simulink model "Vehicle_Radar_Model"  (R2013a)
settings: Solver=ode4  StartTime=0.0  StopTime=100  FixedStep=0.001  MaxStep=0.001  RelTol=1e-3
model workspace (MAT data in the model file):
  Fy_Angle = [-20; -16; -14; -12; -10; -9.5; -9; -8.5; -8; -7.5; -7; -6.5; -6; -5.5; -5; -4.5; -4; -3.5; -3; -2.5; -2; -1.5; -1; -0.5; 0; 0.5; 1; 1.5; 2; 2.5; 3; 3.5; 4; 4.5; 5; 5.5; 6; 6.5; 7; 7.5; 8; 8.5; 9; 9.5; 10; 12; 14; 16; 18; 20]
  Fy_W = [1725 3500 6100 6950 9005]
  Fy_Data = [-1523.64 -1531.91 -1546.58 -1574.53 -1631.62 -1653.27 -1678.67 -1707.8 -1740.18 -1775.12 -1810.95 -1845.3 ... (250 elements, 50x5)]
  Cr = 38255
  Cf = 38925
  lr = 1.6662
  Izz = 4192
  lf = 1.11
  m = 1530
  GearRatio = 17.25
  Pb2Tq_r = 150
  Pb2Tq_f = 300
  t2e = 2000
  R_Tire = 0.33
  Iyy_Tire = 0.9
  Fx_SL = [-1; -0.9; -0.8; -0.7; -0.6; -0.5; -0.4; -0.3; -0.25; -0.2; -0.18; -0.16; -0.14; -0.12; -0.1; -0.08; -0.06; -0.04; -0.02; 0; 0.02; 0.04; 0.06; 0.08; 0.1; 0.12; 0.14; 0.16; 0.18; 0.2; 0.25; 0.3; 0.4; 0.5; 0.6; 0.7; 0.8; 0.9; 1]
  Fx_W = [2105 3995 6120 7900 10100]
  Fx_Data = [-2029.26  -4058.51  -6087.76  -8117.01  -10146.3; -2029.26  -4058.51  -6087.76  -8117.01  -10146.3; -2053.55  -4107.12  -6160.67  -8214.24  -10267.8; -2084.58  -4169.16  -6253.75  -8338.33  -10422.9; -2125.47  -4250.95  -6376.42  -8501.91  -10627.4; -2181.64  -4363.28  -6544.93  -8726.56  -10908.2; -2262.94  -4525.87  -6788.82  -9051.76  -11314.7; -2388.22  -4776.46  -7164.69  -9552.92  -11941.1; -2476.95  -4953.9  -7430.85  -9907.79  -12384.7; -2586.89  -5173.78  -7760.68  -10347.6  -12934.4; -2634.75  -5269.5  -7904.24  -10539  -13173.7; -2680.7  -5361.4  -8042.1  -10722.8  -13403.5; -2717.36  -5434.73  -8152.09  -10869.4  -13586.8; -2729.82  -5459.63  -8189.45  -10919.3  -13649.1; -2689.78  -5379.54  -8069.32  -10759.1  -13448.8; -2548.95  -5097.92  -7646.88  -10195.8  -12744.8; -2240.07  -4480.13  -6720.21  -8960.27  -11200.3; -1701.43  -3402.86  -5104.29  -6805.72  -8507.15; -926.741  -1853.48  -2780.22  -3706.97  -4633.7; 0  0  0  0  0; 926.741  1853.48  2780.22  3706.97  4633.7; 1701.43  3402.86  5104.29  6805.72  8507.15; 2240.07  4480.13  6720.21  8960.27  11200.3; 2548.95  5097.92  7646.88  10195.8  12744.8; 2689.78  5379.54  8069.32  10759.1  13448.8; 2729.82  5459.63  8189.45  10919.3  13649.1; 2717.36  5434.73  8152.09  10869.4  13586.8; 2680.7  5361.4  8042.1  10722.8  13403.5; 2634.75  5269.5  7904.24  10539  13173.7; 2586.89  5173.78  7760.68  10347.6  12934.4; 2476.95  4953.9  7430.85  9907.79  12384.7; 2388.22  4776.46  7164.69  9552.92  11941.1; 2262.94  4525.87  6788.82  9051.76  11314.7; 2181.64  4363.28  6544.93  8726.56  10908.2; 2125.47  4250.95  6376.42  8501.91  10627.4; 2084.58  4169.16  6253.75  8338.33  10422.9; 2053.55  4107.12  6160.67  8214.24  10267.8; 2029.26  4058.51  6087.76  8117.01  10146.3; 2029.26  4058.51  6087.76  8117.01  10146.3]
  g = 9.81
  K = 19
  mu = 0.9
libraries: simulink x1
settings Model: Creator=Park  LastModifiedBy=IVDL
settings DataIOCC: LimitDataPoints=off  SignalLoggingSaveFormat=ModelDataLogs
settings OptimizationCC: ExpressionDepthLimit=2147483647
settings DebuggingCC: MultiTaskDSMMsg=warning  MultiTaskCondExecSysMsg=none  FcnCallInpInsideContextMsg=UseLocalSettings  StrictBusMsg=None
settings RTWCC: IncludeERTFirstTime=on
settings GRTTargetCC: CodeReplacementLibrary=None  CombineOutputUpdateFcns=off  CPPClassGenCompliant=on  GRTInterface=on

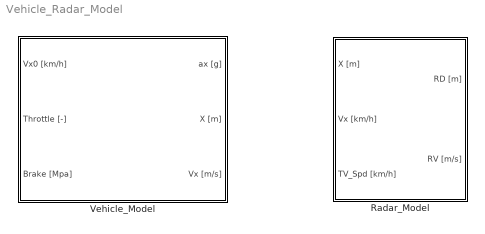
== system Vehicle_Radar_Model ==
  Radar_Model : Subsystem
  Vehicle_Model : Subsystem

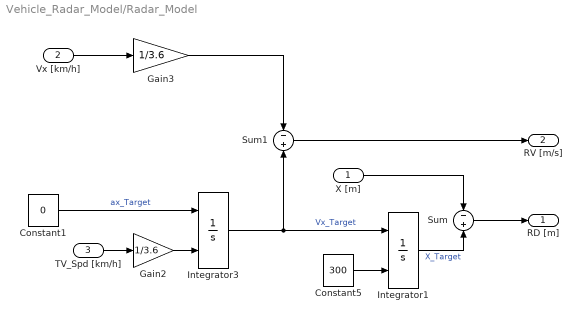
== system Vehicle_Radar_Model/Radar_Model ==
  X [m] : Inport
  Vx [km/h] : Inport  Port=2
  TV_Spd [km/h] : Inport  Port=3
  Constant1 : Constant  Value=0
  Constant5 : Constant  Value=300
  Gain2 : Gain  Gain=1/3.6
  Gain3 : Gain  Gain=1/3.6
  Integrator1 : Integrator  InitialConditionSource=external  InitialCondition=500
  Integrator3 : Integrator  InitialConditionSource=external  InitialCondition=80  LimitOutput=on  LowerSaturationLimit=0
  Sum : Sum  Inputs=-+
  Sum1 : Sum  Inputs=-+
  RD [m] : Outport
  RV [m/s] : Outport  Port=2
  wires:
  TV_Spd [km/h]/1 -> Gain2/1
  Constant1/1 -> Integrator3/1  "ax_Target"
  Integrator3/1 -> Integrator1/1, Sum1/2  "Vx_Target"
  Integrator1/1 -> Sum/2  "X_Target"
  Constant5/1 -> Integrator1/2
  Sum/1 -> RD [m]/1
  X [m]/1 -> Sum/1
  Vx [km/h]/1 -> Gain3/1
  Sum1/1 -> RV [m/s]/1
  Gain2/1 -> Integrator3/2
  Gain3/1 -> Sum1/1

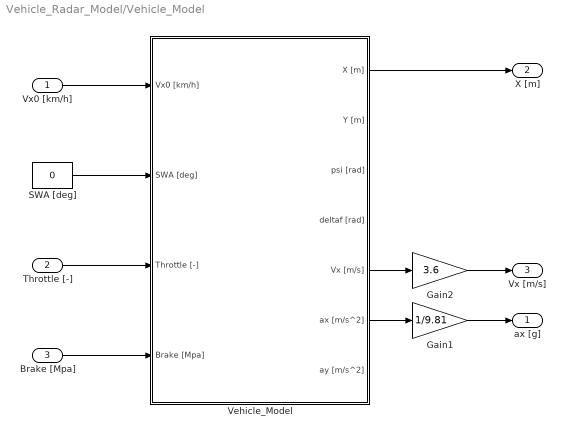
== system Vehicle_Radar_Model/Vehicle_Model ==
  Vx0 [km/h] : Inport
  Throttle [-] : Inport  Port=2
  Brake [Mpa] : Inport  Port=3
  Gain1 : Gain  Gain=1/9.81
  Gain2 : Gain  Gain=3.6
  SWA [deg] : Constant  Value=0
  Vehicle_Model : Subsystem
  ax [g] : Outport
  X [m] : Outport  Port=2
  Vx [m/s] : Outport  Port=3
  wires:
  Gain1/1 -> ax [g]/1
  Gain2/1 -> Vx [m/s]/1
  Vehicle_Model/1(X [m]) -> X [m]/1
  Throttle [-]/1 -> Vehicle_Model/3(Throttle [-])
  Brake [Mpa]/1 -> Vehicle_Model/4(Brake [Mpa])
  Vehicle_Model/6(ax [m/s^2]) -> Gain1/1
  Vehicle_Model/5(Vx [m/s]) -> Gain2/1
  SWA [deg]/1 -> Vehicle_Model/2(SWA [deg])
  Vx0 [km/h]/1 -> Vehicle_Model/1(Vx0 [km/h])

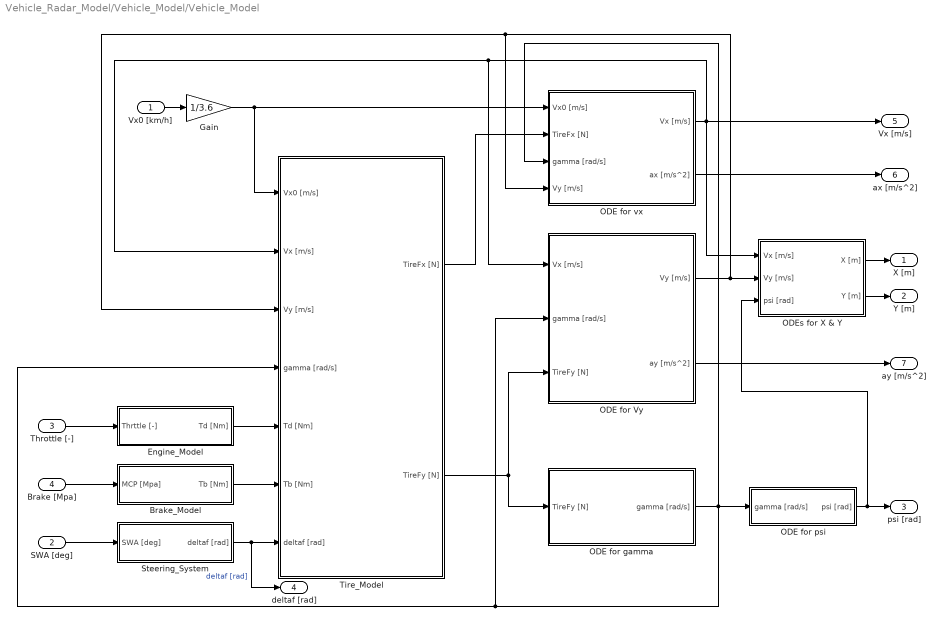
== system Vehicle_Radar_Model/Vehicle_Model/Vehicle_Model ==
  Vx0 [km/h] : Inport
  SWA [deg] : Inport  Port=2
  Throttle [-] : Inport  Port=3
  Brake [Mpa] : Inport  Port=4
  Brake_Model : Subsystem
  Engine_Model : Subsystem
  Gain : Gain  Gain=1/3.6
  ODE for Vy : Subsystem
  ODE for gamma : Subsystem
  ODE for psi : Subsystem
  ODE for vx : Subsystem
  ODEs for X & Y : Subsystem
  Steering_System : Subsystem
  Tire_Model : Subsystem
  X [m] : Outport
  Y [m] : Outport  Port=2
  psi [rad] : Outport  Port=3
  deltaf [rad] : Outport  Port=4
  Vx [m/s] : Outport  Port=5
  ax [m/s^2] : Outport  Port=6
  ay [m/s^2] : Outport  Port=7
  wires:
  ODE for Vy/2(ay [m/s^2]) -> ay [m/s^2]/1
  ODE for vx/2(ax [m/s^2]) -> ax [m/s^2]/1
  ODEs for X & Y/2(Y [m]) -> Y [m]/1
  ODEs for X & Y/1(X [m]) -> X [m]/1
  ODE for psi/1(psi [rad]) -> ODEs for X & Y/3(psi [rad]), psi [rad]/1
  ODE for Vy/1(Vy [m/s]) -> ODEs for X & Y/2(Vy [m/s]), Tire_Model/3(Vy [m/s]), ODE for vx/4(Vy [m/s])
  ODE for gamma/1(gamma [rad/s]) -> ODE for Vy/2(gamma [rad/s]), Tire_Model/4(gamma [rad/s]), ODE for psi/1(gamma [rad/s]), ODE for vx/3(gamma [rad/s])
  Tire_Model/2(TireFy [N]) -> ODE for gamma/1(TireFy [N]), ODE for Vy/3(TireFy [N])
  ODE for vx/1(Vx [m/s]) -> Tire_Model/2(Vx [m/s]), ODE for Vy/1(Vx [m/s]), ODEs for X & Y/1(Vx [m/s]), Vx [m/s]/1
  Steering_System/1(deltaf [rad]) -> Tire_Model/7(deltaf [rad]), deltaf [rad]/1  "deltaf [rad]"
  Tire_Model/1(TireFx [N]) -> ODE for vx/2(TireFx [N])
  Throttle [-]/1 -> Engine_Model/1(Thrttle [-])
  Brake [Mpa]/1 -> Brake_Model/1(MCP [Mpa])
  Brake_Model/1(Tb [Nm]) -> Tire_Model/6(Tb [Nm])
  Engine_Model/1(Td [Nm]) -> Tire_Model/5(Td [Nm])
  Gain/1 -> Tire_Model/1(Vx0 [m/s]), ODE for vx/1(Vx0 [m/s])
  SWA [deg]/1 -> Steering_System/1(SWA [deg])
  Vx0 [km/h]/1 -> Gain/1

== system Vehicle_Radar_Model/Vehicle_Model/Vehicle_Model/Brake_Model ==
  MCP [Mpa] : Inport
  Gain : Gain  Gain=2*Pb2Tq_f
  Gain1 : Gain  Gain=2*Pb2Tq_r
  Mux : Mux  Inputs=2
  Transfer Fcn : TransferFcn  Denominator=[0.06 1]
  Transfer Fcn1 : TransferFcn  Denominator=[0.06 1]
  Tb [Nm] : Outport
  wires:
  Transfer Fcn1/1 -> Mux/2
  Transfer Fcn/1 -> Mux/1
  Mux/1 -> Tb [Nm]/1
  MCP [Mpa]/1 -> Gain/1, Gain1/1
  Gain1/1 -> Transfer Fcn1/1  "Tb_r [Nm]"
  Gain/1 -> Transfer Fcn/1  "Tb_f [Nm]"

== system Vehicle_Radar_Model/Vehicle_Model/Vehicle_Model/Engine_Model ==
  Thrttle [-] : Inport
  Gain : Gain  Gain=t2e
  Transfer Fcn : TransferFcn  Numerator=[100]  Denominator=[1 2*0.5*10 100]
  Td [Nm] : Outport
  wires:
  Transfer Fcn/1 -> Td [Nm]/1
  Gain/1 -> Transfer Fcn/1
  Thrttle [-]/1 -> Gain/1

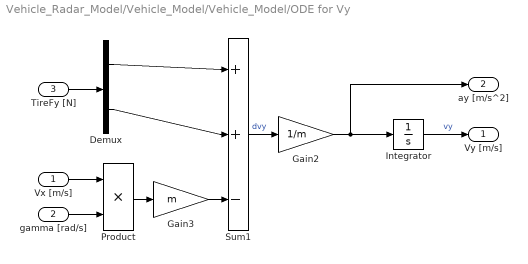
== system Vehicle_Radar_Model/Vehicle_Model/Vehicle_Model/ODE for Vy ==
  Vx [m/s] : Inport
  gamma [rad/s] : Inport  Port=2
  TireFy [N] : Inport  Port=3
  Demux : Demux  Outputs=2
  Gain2 : Gain  Gain=1/m
  Gain3 : Gain  Gain=m
  Integrator : Integrator
  Product : Product  RndMeth=Zero
  Sum1 : Sum  Inputs=++|-
  Vy [m/s] : Outport
  ay [m/s^2] : Outport  Port=2
  wires:
  Gain2/1 -> Integrator/1, ay [m/s^2]/1
  Gain3/1 -> Sum1/3
  TireFy [N]/1 -> Demux/1
  gamma [rad/s]/1 -> Product/2
  Vx [m/s]/1 -> Product/1
  Integrator/1 -> Vy [m/s]/1  "vy"
  Product/1 -> Gain3/1
  Sum1/1 -> Gain2/1  "dvy"
  Demux/2 -> Sum1/2
  Demux/1 -> Sum1/1

== system Vehicle_Radar_Model/Vehicle_Model/Vehicle_Model/ODE for gamma ==
  TireFy [N] : Inport
  Demux : Demux  Outputs=2
  Gain4 : Gain  Gain=1/Izz
  Gain5 : Gain  Gain=lf
  Gain6 : Gain  Gain=lr
  Integrator2 : Integrator
  Sum2 : Sum  Inputs=+-
  gamma [rad/s] : Outport
  wires:
  TireFy [N]/1 -> Demux/1
  Demux/2 -> Gain6/1
  Integrator2/1 -> gamma [rad/s]/1  "gamma"
  Demux/1 -> Gain5/1
  Gain6/1 -> Sum2/2
  Gain5/1 -> Sum2/1
  Gain4/1 -> Integrator2/1
  Sum2/1 -> Gain4/1

== system Vehicle_Radar_Model/Vehicle_Model/Vehicle_Model/ODE for psi ==
  gamma [rad/s] : Inport
  Integrator : Integrator  ContinuousStateAttributes='psi'
  psi [rad] : Outport
  wires:
  gamma [rad/s]/1 -> Integrator/1  "dpsi"
  Integrator/1 -> psi [rad]/1

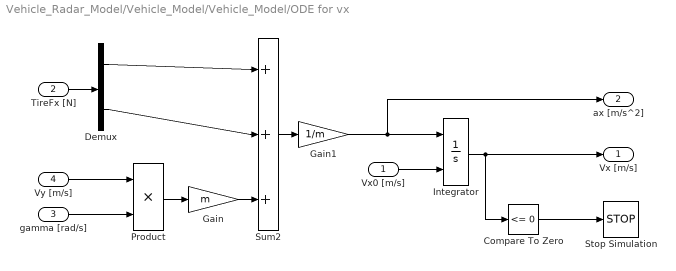
== system Vehicle_Radar_Model/Vehicle_Model/Vehicle_Model/ODE for vx ==
  Vx0 [m/s] : Inport
  TireFx [N] : Inport  Port=2
  gamma [rad/s] : Inport  Port=3
  Vy [m/s] : Inport  Port=4
  Compare To Zero : simulink/Logic and Bit Operations/Compare To Zero  relop=<=  OutDataTypeStr=boolean
  Demux : Demux  Outputs=2
  Gain : Gain  Gain=m
  Gain1 : Gain  Gain=1/m
  Integrator : Integrator  InitialConditionSource=external
  Product : Product  RndMeth=Zero
  Stop Simulation : Stop
  Sum2 : Sum  Inputs=++|+
  Vx [m/s] : Outport
  ax [m/s^2] : Outport  Port=2
  wires:
  Gain1/1 -> Integrator/1, ax [m/s^2]/1
  Compare To Zero/1 -> Stop Simulation/1
  Gain/1 -> Sum2/3
  Product/1 -> Gain/1
  Sum2/1 -> Gain1/1
  gamma [rad/s]/1 -> Product/2
  Vy [m/s]/1 -> Product/1
  Demux/2 -> Sum2/2
  Demux/1 -> Sum2/1
  TireFx [N]/1 -> Demux/1
  Integrator/1 -> Vx [m/s]/1, Compare To Zero/1
  Vx0 [m/s]/1 -> Integrator/2

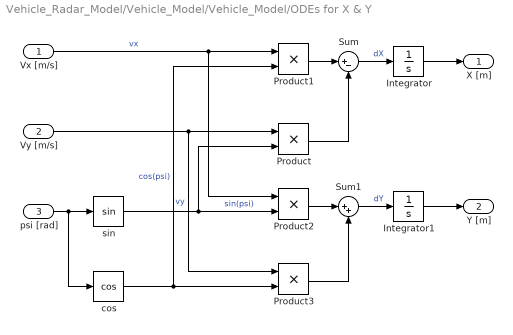
== system Vehicle_Radar_Model/Vehicle_Model/Vehicle_Model/ODEs for X & Y ==
  Vx [m/s] : Inport
  Vy [m/s] : Inport  Port=2
  psi [rad] : Inport  Port=3
  Integrator : Integrator  ContinuousStateAttributes='X'
  Integrator1 : Integrator  ContinuousStateAttributes='Y'
  Product{,1..3} (4 alike) : Product  RndMeth=Zero
  Sum : Sum  Inputs=|+-
  Sum1 : Sum  Inputs=|++
  cos : Trigonometry  Operator=cos
  sin : Trigonometry
  X [m] : Outport
  Y [m] : Outport  Port=2
  wires:
  Integrator1/1 -> Y [m]/1
  Integrator/1 -> X [m]/1
  Sum1/1 -> Integrator1/1  "dY"
  Product3/1 -> Sum1/2
  Product2/1 -> Sum1/1
  Sum/1 -> Integrator/1  "dX"
  Product/1 -> Sum/2
  Product1/1 -> Sum/1
  cos/1 -> Product3/2, Product1/2  "cos(psi)"
  Vx [m/s]/1 -> Product2/1, Product1/1  "vx"
  Vy [m/s]/1 -> Product3/1, Product/1  "vy"
  sin/1 -> Product2/2, Product/2  "sin(psi)"
  psi [rad]/1 -> cos/1, sin/1

== system Vehicle_Radar_Model/Vehicle_Model/Vehicle_Model/Steering_System ==
  SWA [deg] : Inport
  Gain : Gain  Gain=1/GearRatio
  Gain5 : Gain  Gain=pi/180
  Saturation : Saturate  UpperLimit=540  LowerLimit=-540
  deltaf [rad] : Outport
  wires:
  Saturation/1 -> Gain/1
  SWA [deg]/1 -> Saturation/1
  Gain5/1 -> deltaf [rad]/1
  Gain/1 -> Gain5/1

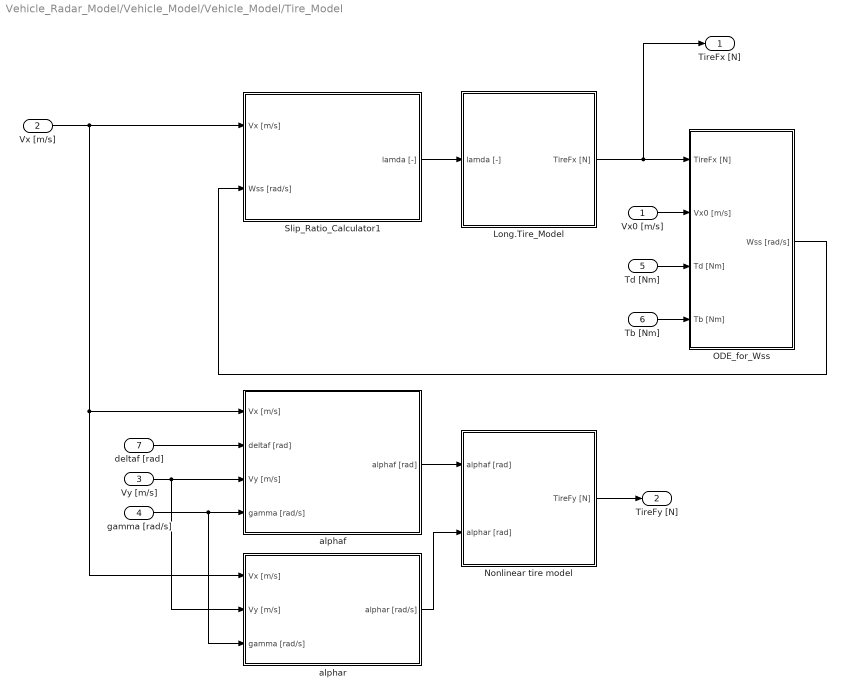
== system Vehicle_Radar_Model/Vehicle_Model/Vehicle_Model/Tire_Model ==
  Vx0 [m/s] : Inport
  Vx [m/s] : Inport  Port=2
  Vy [m/s] : Inport  Port=3
  gamma [rad/s] : Inport  Port=4
  Td [Nm] : Inport  Port=5
  Tb [Nm] : Inport  Port=6
  deltaf [rad] : Inport  Port=7
  Long.Tire_Model : Subsystem
  Nonlinear tire model : Subsystem
  ODE_for_Wss : Subsystem
  Slip_Ratio_Calculator1 : Subsystem
  alphaf : Subsystem
  alphar : Subsystem
  TireFx [N] : Outport
  TireFy [N] : Outport  Port=2
  wires:
  Nonlinear tire model/1(TireFy [N]) -> TireFy [N]/1
  gamma [rad/s]/1 -> alphaf/4(gamma [rad/s]), alphar/3(gamma [rad/s])
  Vy [m/s]/1 -> alphar/2(Vy [m/s]), alphaf/3(Vy [m/s])
  deltaf [rad]/1 -> alphaf/2(deltaf [rad])
  alphar/1(alphar [rad/s]) -> Nonlinear tire model/2(alphar [rad])
  alphaf/1(alphaf [rad]) -> Nonlinear tire model/1(alphaf [rad])
  ODE_for_Wss/1(Wss [rad/s]) -> Slip_Ratio_Calculator1/2(Wss [rad/s])
  Tb [Nm]/1 -> ODE_for_Wss/4(Tb [Nm])
  Td [Nm]/1 -> ODE_for_Wss/3(Td [Nm])
  Vx0 [m/s]/1 -> ODE_for_Wss/2(Vx0 [m/s])
  Vx [m/s]/1 -> alphaf/1(Vx [m/s]), alphar/1(Vx [m/s]), Slip_Ratio_Calculator1/1(Vx [m/s])
  Slip_Ratio_Calculator1/1(lamda [-]) -> Long.Tire_Model/1(lamda [-])
  Long.Tire_Model/1(TireFx [N]) -> ODE_for_Wss/1(TireFx [N]), TireFx [N]/1

== system Vehicle_Radar_Model/Vehicle_Model/Vehicle_Model/Tire_Model/Long.Tire_Model ==
  lamda [-] : Inport
  Demux : Demux  Outputs=2
  Fx_f_Calculator : Subsystem
  Fx_r_Calculator : Subsystem
  Mux : Mux  Inputs=2
  TireFx [N] : Outport
  wires:
  Mux/1 -> TireFx [N]/1
  Fx_r_Calculator/1(TireFx _r [N]) -> Mux/2
  Fx_f_Calculator/1(TireFx _f [N]) -> Mux/1
  Demux/2 -> Fx_r_Calculator/1(lamda_r [-])
  Demux/1 -> Fx_f_Calculator/1(lamda_f [-])
  lamda [-]/1 -> Demux/1

== system Vehicle_Radar_Model/Vehicle_Model/Vehicle_Model/Tire_Model/Nonlinear tire model ==
  alphaf [rad] : Inport
  alphar [rad] : Inport  Port=2
  Gain : Gain  Gain=-2*Cf*mu/K
  Gain1 : Gain  Gain=-2*Cr*mu/K
  Gain2 : Gain  Gain=K/mu
  Gain3 : Gain  Gain=K/mu
  Mux : Mux  Inputs=2
  atan : Trigonometry  Operator=atan
  atan1 : Trigonometry  Operator=atan
  TireFy [N] : Outport
  wires:
  Gain/1 -> Mux/1
  Gain1/1 -> Mux/2
  alphar [rad]/1 -> Gain3/1
  alphaf [rad]/1 -> Gain2/1
  atan1/1 -> Gain1/1
  Gain3/1 -> atan1/1
  atan/1 -> Gain/1
  Gain2/1 -> atan/1
  Mux/1 -> TireFy [N]/1

== system Vehicle_Radar_Model/Vehicle_Model/Vehicle_Model/Tire_Model/ODE_for_Wss ==
  TireFx [N] : Inport
  Vx0 [m/s] : Inport  Port=2
  Td [Nm] : Inport  Port=3
  Tb [Nm] : Inport  Port=4
  Demux : Demux  Outputs=2
  Demux1 : Demux  Outputs=2
  Mux : Mux  Inputs=2
  ODE_for_Wss_f : Subsystem
  ODE_for_Wss_r : Subsystem
  Wss [rad/s] : Outport
  wires:
  Mux/1 -> Wss [rad/s]/1
  ODE_for_Wss_r/1(Wss_r [rad/s]) -> Mux/2
  ODE_for_Wss_f/1(Wss_f [rad/s]) -> Mux/1
  Demux1/2 -> ODE_for_Wss_r/2(TireFx _r [N])  "TireFx _r [N]"
  TireFx [N]/1 -> Demux1/1
  Demux/2 -> ODE_for_Wss_r/3(Tb_r [Nm])
  Demux/1 -> ODE_for_Wss_f/4(Tb_f [Nm])
  Tb [Nm]/1 -> Demux/1
  Vx0 [m/s]/1 -> ODE_for_Wss_f/2(Vx0 [m/s]), ODE_for_Wss_r/1(Vx0 [m/s])
  Td [Nm]/1 -> ODE_for_Wss_f/1(Td_f [Nm])
  Demux1/1 -> ODE_for_Wss_f/3(TireFx _f [N])  "TireFx _f [N]"

== system Vehicle_Radar_Model/Vehicle_Model/Vehicle_Model/Tire_Model/Slip_Ratio_Calculator1 ==
  Vx [m/s] : Inport
  Wss [rad/s] : Inport  Port=2
  Demux : Demux  Outputs=2
  Mux : Mux  Inputs=2
  lamda_f_Calculator : Subsystem
  lamda_r_Calculator : Subsystem
  lamda [-] : Outport
  wires:
  Demux/2 -> lamda_r_Calculator/1(Wss_r [rad/s])  "Wss_r [rad/s]"
  Demux/1 -> lamda_f_Calculator/1(Wss_f [rad/s])  "Wss_f [rad/s]"
  Wss [rad/s]/1 -> Demux/1
  Mux/1 -> lamda [-]/1
  lamda_r_Calculator/1(lamda_f [-]) -> Mux/2  "lamda_r [-]"
  lamda_f_Calculator/1(lamda_f [-]) -> Mux/1  "lamda_f [-]"
  Vx [m/s]/1 -> lamda_r_Calculator/2(Vx [m/s]), lamda_f_Calculator/2(Vx [m/s])

== system Vehicle_Radar_Model/Vehicle_Model/Vehicle_Model/Tire_Model/alphaf ==
  Vx [m/s] : Inport
  deltaf [rad] : Inport  Port=2
  Vy [m/s] : Inport  Port=3
  gamma [rad/s] : Inport  Port=4
  Divide : Product  Inputs=*/
  Gain : Gain  Gain=lf
  Sum : Sum  Inputs=++|
  Sum1 : Sum  Inputs=|+-
  Trigonometric Function : Trigonometry  Operator=atan
  alphaf [rad] : Outport
  wires:
  Sum1/1 -> alphaf [rad]/1
  deltaf [rad]/1 -> Sum1/2
  Trigonometric Function/1 -> Sum1/1
  Divide/1 -> Trigonometric Function/1
  Vx [m/s]/1 -> Divide/2
  Sum/1 -> Divide/1
  Gain/1 -> Sum/2
  Vy [m/s]/1 -> Sum/1
  gamma [rad/s]/1 -> Gain/1

== system Vehicle_Radar_Model/Vehicle_Model/Vehicle_Model/Tire_Model/alphar ==
  Vx [m/s] : Inport
  Vy [m/s] : Inport  Port=2
  gamma [rad/s] : Inport  Port=3
  Divide : Product  Inputs=*/
  Gain : Gain  Gain=lr
  Sum : Sum  Inputs=+-|
  Trigonometric Function : Trigonometry  Operator=atan
  alphar [rad/s] : Outport
  wires:
  gamma [rad/s]/1 -> Gain/1
  Vy [m/s]/1 -> Sum/1
  Gain/1 -> Sum/2
  Sum/1 -> Divide/1
  Vx [m/s]/1 -> Divide/2
  Divide/1 -> Trigonometric Function/1
  Trigonometric Function/1 -> alphar [rad/s]/1

== system Vehicle_Radar_Model/Vehicle_Model/Vehicle_Model/Tire_Model/Long.Tire_Model/Fx_f_Calculator ==
  lamda_f [-] : Inport
  Constant : Constant  Value=m*9.81
  Fx_Table_fl : Lookup2D  RowIndex=Fx_SL  ColumnIndex=Fx_W  Table=Fx_Data  SaturateOnIntegerOverflow=on
  Gain : Gain  Gain=lr / (lf+lr)
  Gain1 : Gain  Gain=2
  Gain4 : Gain  Gain=0.5
  TireFx _f [N] : Outport
  wires:
  Fx_Table_fl/1 -> Gain1/1
  Gain4/1 -> Fx_Table_fl/2  "Wf [N]"
  Gain/1 -> Gain4/1
  Constant/1 -> Gain/1
  lamda_f [-]/1 -> Fx_Table_fl/1
  Gain1/1 -> TireFx _f [N]/1

== system Vehicle_Radar_Model/Vehicle_Model/Vehicle_Model/Tire_Model/Long.Tire_Model/Fx_r_Calculator ==
  lamda_r [-] : Inport
  Constant1 : Constant  Value=m*9.81
  Fx_Table_fl1 : Lookup2D  RowIndex=Fx_SL  ColumnIndex=Fx_W  Table=Fx_Data  SaturateOnIntegerOverflow=on
  Gain2 : Gain  Gain=lf / (lf+lr)
  Gain3 : Gain  Gain=2
  Gain5 : Gain  Gain=0.5
  TireFx _r [N] : Outport
  wires:
  Gain3/1 -> TireFx _r [N]/1
  Gain5/1 -> Fx_Table_fl1/2  "Wr [N]"
  Gain2/1 -> Gain5/1
  Fx_Table_fl1/1 -> Gain3/1
  Constant1/1 -> Gain2/1
  lamda_r [-]/1 -> Fx_Table_fl1/1

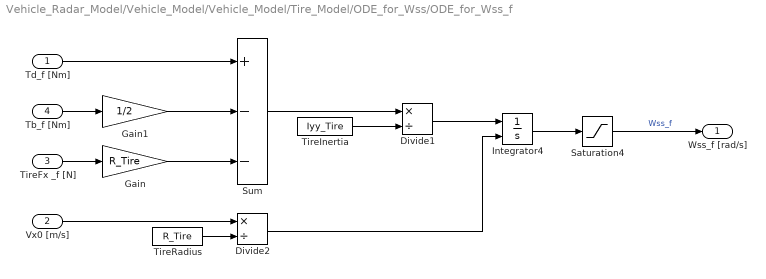
== system Vehicle_Radar_Model/Vehicle_Model/Vehicle_Model/Tire_Model/ODE_for_Wss/ODE_for_Wss_f ==
  Td_f [Nm] : Inport
  Vx0 [m/s] : Inport  Port=2
  TireFx _f [N] : Inport  Port=3
  Tb_f [Nm] : Inport  Port=4
  Divide1 : Product  Inputs=*/
  Divide2 : Product  Inputs=*/
  Gain : Gain  Gain=R_Tire
  Gain1 : Gain  Gain=1/2
  Integrator4 : Integrator  InitialConditionSource=external
  Saturation4 : Saturate  UpperLimit=255  LowerLimit=0
  Sum : Sum  Inputs=+--
  TireInertia : Constant  Value=Iyy_Tire
  TireRadius : Constant  Value=R_Tire
  Wss_f [rad/s] : Outport
  wires:
  Gain1/1 -> Sum/2
  Saturation4/1 -> Wss_f [rad/s]/1  "Wss_f"
  Integrator4/1 -> Saturation4/1
  Divide2/1 -> Integrator4/2
  Vx0 [m/s]/1 -> Divide2/1
  TireRadius/1 -> Divide2/2
  Divide1/1 -> Integrator4/1
  TireInertia/1 -> Divide1/2
  Sum/1 -> Divide1/1
  TireFx _f [N]/1 -> Gain/1
  Tb_f [Nm]/1 -> Gain1/1
  Td_f [Nm]/1 -> Sum/1
  Gain/1 -> Sum/3

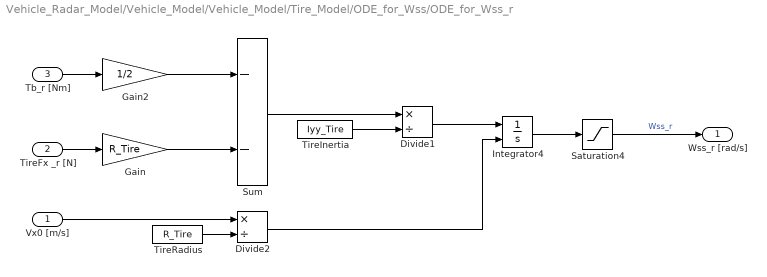
== system Vehicle_Radar_Model/Vehicle_Model/Vehicle_Model/Tire_Model/ODE_for_Wss/ODE_for_Wss_r ==
  Vx0 [m/s] : Inport
  TireFx _r [N] : Inport  Port=2
  Tb_r [Nm] : Inport  Port=3
  Divide1 : Product  Inputs=*/
  Divide2 : Product  Inputs=*/
  Gain : Gain  Gain=R_Tire
  Gain2 : Gain  Gain=1/2
  Integrator4 : Integrator  InitialConditionSource=external
  Saturation4 : Saturate  UpperLimit=255  LowerLimit=0
  Sum : Sum  Inputs=--
  TireInertia : Constant  Value=Iyy_Tire
  TireRadius : Constant  Value=R_Tire
  Wss_r [rad/s] : Outport
  wires:
  Gain2/1 -> Sum/1
  Gain/1 -> Sum/2
  Tb_r [Nm]/1 -> Gain2/1
  TireFx _r [N]/1 -> Gain/1
  Sum/1 -> Divide1/1
  TireInertia/1 -> Divide1/2
  Divide1/1 -> Integrator4/1
  TireRadius/1 -> Divide2/2
  Vx0 [m/s]/1 -> Divide2/1
  Divide2/1 -> Integrator4/2
  Integrator4/1 -> Saturation4/1
  Saturation4/1 -> Wss_r [rad/s]/1  "Wss_r"

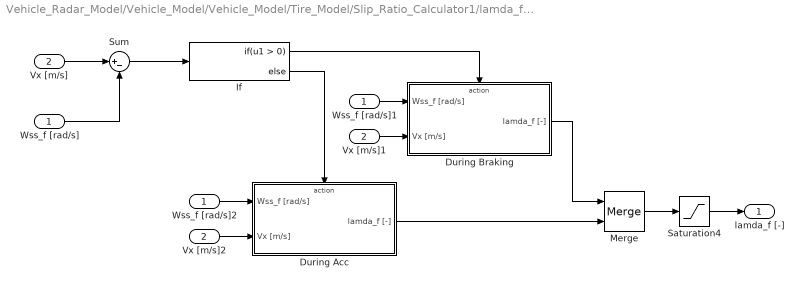
== system Vehicle_Radar_Model/Vehicle_Model/Vehicle_Model/Tire_Model/Slip_Ratio_Calculator1/lamda_f_Calculator ==
  Wss_f [rad/s] : Inport
  Vx [m/s] : Inport  Port=2
  During Acc : Subsystem
  During Braking : Subsystem
  If : If
  Merge : Merge
  Saturation4 : Saturate  UpperLimit=1  LowerLimit=-1
  Sum : Sum  Inputs=|+-
  Vx [m/s]1 : InportShadow  Port=2
  Vx [m/s]2 : InportShadow  Port=2
  Wss_f [rad/s]1 : InportShadow
  Wss_f [rad/s]2 : InportShadow
  lamda_f [-] : Outport
  wires:
  Saturation4/1 -> lamda_f [-]/1
  Vx [m/s]2/1 -> During Acc/2(Vx [m/s])
  Wss_f [rad/s]2/1 -> During Acc/1(Wss_f [rad/s])
  Wss_f [rad/s]1/1 -> During Braking/1(Wss_f [rad/s])
  Vx [m/s]1/1 -> During Braking/2(Vx [m/s])
  Sum/1 -> If/1
  Vx [m/s]/1 -> Sum/1
  Wss_f [rad/s]/1 -> Sum/2
  During Braking/1(lamda_f [-]) -> Merge/1
  During Acc/1(lamda_f [-]) -> Merge/2
  Merge/1 -> Saturation4/1
  If/2 -> During Acc/Action
  If/1 -> During Braking/Action

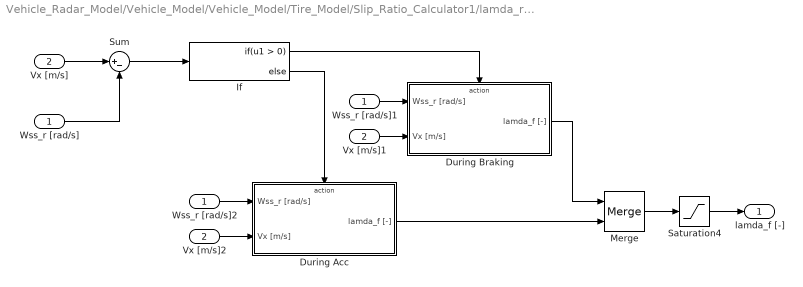
== system Vehicle_Radar_Model/Vehicle_Model/Vehicle_Model/Tire_Model/Slip_Ratio_Calculator1/lamda_r_Calculator ==
  Wss_r [rad/s] : Inport
  Vx [m/s] : Inport  Port=2
  During Acc : Subsystem
  During Braking : Subsystem
  If : If
  Merge : Merge
  Saturation4 : Saturate  UpperLimit=1  LowerLimit=-1
  Sum : Sum  Inputs=|+-
  Vx [m/s]1 : InportShadow  Port=2
  Vx [m/s]2 : InportShadow  Port=2
  Wss_r [rad/s]1 : InportShadow
  Wss_r [rad/s]2 : InportShadow
  lamda_f [-] : Outport
  wires:
  If/1 -> During Braking/Action
  If/2 -> During Acc/Action
  Merge/1 -> Saturation4/1
  During Acc/1(lamda_f [-]) -> Merge/2
  During Braking/1(lamda_f [-]) -> Merge/1
  Wss_r [rad/s]/1 -> Sum/2
  Vx [m/s]/1 -> Sum/1
  Sum/1 -> If/1
  Vx [m/s]1/1 -> During Braking/2(Vx [m/s])
  Wss_r [rad/s]1/1 -> During Braking/1(Wss_r [rad/s])
  Wss_r [rad/s]2/1 -> During Acc/1(Wss_r [rad/s])
  Vx [m/s]2/1 -> During Acc/2(Vx [m/s])
  Saturation4/1 -> lamda_f [-]/1

== system Vehicle_Radar_Model/Vehicle_Model/Vehicle_Model/Tire_Model/Slip_Ratio_Calculator1/lamda_f_Calculator/During Acc ==
  note: Slip Ratio During Acc.
  note: (Rw-Vx) / Rw
  Wss_f [rad/s] : Inport
  Vx [m/s] : Inport  Port=2
  Action Port : ActionPort  ActionType=else
  Divide : Product  Inputs=*/
  Product2 : Product  RndMeth=Zero
  Subtract : Sum  Inputs=-+
  TireRadius : Constant  Value=R_Tire
  lamda_f [-] : Outport
  wires:
  Subtract/1 -> Divide/1
  Divide/1 -> lamda_f [-]/1
  Vx [m/s]/1 -> Subtract/1
  Wss_f [rad/s]/1 -> Product2/1
  TireRadius/1 -> Product2/2
  Product2/1 -> Subtract/2, Divide/2

== system Vehicle_Radar_Model/Vehicle_Model/Vehicle_Model/Tire_Model/Slip_Ratio_Calculator1/lamda_f_Calculator/During Braking ==
  Wss_f [rad/s] : Inport
  Vx [m/s] : Inport  Port=2
  Action Port : ActionPort  ActionType=then
  Divide : Product  Inputs=/*
  Gain : Gain  Gain=-1
  Product2 : Product  RndMeth=Zero
  Subtract : Sum  Inputs=+-
  TireRadius : Constant  Value=R_Tire
  lamda_f [-] : Outport
  wires:
  Gain/1 -> lamda_f [-]/1
  Divide/1 -> Gain/1
  Subtract/1 -> Divide/2
  Product2/1 -> Subtract/2
  TireRadius/1 -> Product2/2
  Wss_f [rad/s]/1 -> Product2/1
  Vx [m/s]/1 -> Divide/1, Subtract/1

== system Vehicle_Radar_Model/Vehicle_Model/Vehicle_Model/Tire_Model/Slip_Ratio_Calculator1/lamda_r_Calculator/During Acc ==
  note: (Rw-Vx) / Rw
  note: Slip Ratio During Acc.
  Wss_r [rad/s] : Inport
  Vx [m/s] : Inport  Port=2
  Action Port : ActionPort  ActionType=else
  Divide : Product  Inputs=*/
  Product2 : Product  RndMeth=Zero
  Subtract : Sum  Inputs=-+
  TireRadius : Constant  Value=R_Tire
  lamda_f [-] : Outport
  wires:
  Product2/1 -> Divide/2, Subtract/2
  TireRadius/1 -> Product2/2
  Wss_r [rad/s]/1 -> Product2/1
  Vx [m/s]/1 -> Subtract/1
  Divide/1 -> lamda_f [-]/1
  Subtract/1 -> Divide/1

== system Vehicle_Radar_Model/Vehicle_Model/Vehicle_Model/Tire_Model/Slip_Ratio_Calculator1/lamda_r_Calculator/During Braking ==
  note: (Rw-Vx) / Vx
  note: Slip Ratio During Braking
  Wss_r [rad/s] : Inport
  Vx [m/s] : Inport  Port=2
  Action Port : ActionPort  ActionType=then
  Divide : Product  Inputs=/*
  Product2 : Product  RndMeth=Zero
  Subtract : Sum  Inputs=-+
  TireRadius : Constant  Value=R_Tire
  lamda_f [-] : Outport
  wires:
  Vx [m/s]/1 -> Subtract/1, Divide/1
  Wss_r [rad/s]/1 -> Product2/1
  TireRadius/1 -> Product2/2
  Product2/1 -> Subtract/2
  Subtract/1 -> Divide/2
  Divide/1 -> lamda_f [-]/1
